simulink library "powerlib_modelsV2"  (Simulink 6.0)
settings: Solver=ode45  SolverMode=SingleTasking  StartTime=0.0  StopTime=10.0  RelTol=1e-3
values from neighbouring files (symbols this model uses):
  Ts = get(handles.edit1,'string')    [powergui.m]
undefined symbols (not defined in the file or in its folder): A, Ac, B, Bc, C, Cc, Cs, Current, damp, Dc, Dd, DiscIntNeverNeededParam, dref, dwo, exc, F, fb, gate, GH, GHd, GI, GId, GL, GLd, H, HT, hyd, ib, ib2, io, isfinite, j, K, Kd, Kg, L, Lad, Laq, lim, LIM, Ll, Llfd, Llkd, Llkq1, Llkq2, Llr, Lls, LowerFlux, N, N2, Nb, Nb2, nb_arm, p, Par_HarmoA_pu, Par_HarmoB_pu, Par_Timing_Harmo, Par_Timing_Variation, Par_Vps, Pb ... (+57)
libraries: powerlib_extras x14
(part 11 of 11)

== system powerlib_modelsV2/Discrete/asynchronous_machine/abc2qd/Rotor reference frame ==
  In1 : Inport  Port=1  LatchInput=off
  Enable : EnablePort  StatesWhenEnabling=reset
  Mux2 : Mux  Inputs=2
  Mux3 : Mux  Inputs=2
  vdr : Fcn  Expr=-sqrt3_3 * u[2]
  vds : Fcn  Expr=one_third * (2*u[5]*u[3] + (u[5]-sqrt3*u[6]) * u[4])
  vqr : Fcn  Expr=one_third * (2*u[1] + u[2])
  vqs : Fcn  Expr=one_third * (2*u[6]*u[3] + (u[6]+sqrt3*u[5]) * u[4])
  vqr,vdr : Outport  OutputWhenDisabled=reset  InitialOutput=0
  vqs,vds : Outport  Port=2  OutputWhenDisabled=reset  InitialOutput=0
  wires:
  In1/1 -> vdr/1, vds/1, vqs/1, vqr/1
  Mux3/1 -> vqr,vdr/1  "Vqr,vdr"
  vqr/1 -> Mux3/1
  vdr/1 -> Mux3/2
  Mux2/1 -> vqs,vds/1  "Vqs,vds"
  vds/1 -> Mux2/2
  vqs/1 -> Mux2/1

== system powerlib_modelsV2/Discrete/asynchronous_machine/abc2qd/Stationary reference frame ==
  In1 : Inport  Port=1  LatchInput=off
  Enable : EnablePort  StatesWhenEnabling=reset
  Mux2 : Mux  Inputs=2
  Mux3 : Mux  Inputs=2
  vdr : Fcn  Expr=one_third * (-2*u[5]*u[1] + (-u[5]-sqrt3*u[6]) * u[2])
  vds : Fcn  Expr=-sqrt3_3*u[4]
  vqr : Fcn  Expr=one_third * (2*u[6]*u[1] + (u[6]-sqrt3*u[5]) * u[2])
  vqs : Fcn  Expr=one_third * (2*u[3] + u[4])
  vqr,vdr : Outport  OutputWhenDisabled=reset  InitialOutput=0
  vqs,vds : Outport  Port=2  OutputWhenDisabled=reset  InitialOutput=0
  wires:
  Mux3/1 -> vqr,vdr/1  "Vqr,vdr"
  In1/1 -> vdr/1, vqs/1, vds/1, vqr/1
  vdr/1 -> Mux3/2
  vqr/1 -> Mux3/1
  Mux2/1 -> vqs,vds/1  "Vqs,vds"
  vqs/1 -> Mux2/1
  vds/1 -> Mux2/2

== system powerlib_modelsV2/Discrete/asynchronous_machine/abc2qd/Synchronous reference frame ==
  In1 : Inport  Port=1  LatchInput=off
  Enable : EnablePort  StatesWhenEnabling=reset
  Mux2 : Mux  Inputs=2
  Mux3 : Mux  Inputs=2
  vdr : Fcn  Expr=(2*u[5]*u[1] + (u[5]-sqrt3*u[6]) * u[2]) / 3
  vds : Fcn  Expr=(2*u[7]*u[3] + (u[7]-sqrt3*u[8]) * u[4]) / 3
  vqr : Fcn  Expr=(2*u[6]*u[1] + (u[6]+sqrt3*u[5]) * u[2]) / 3
  vqs : Fcn  Expr=(2*u[8]*u[3] + (u[8]+sqrt3*u[7]) * u[4]) / 3
  vqr,vdr : Outport  OutputWhenDisabled=reset  InitialOutput=0
  vqs,vds : Outport  Port=2  OutputWhenDisabled=reset  InitialOutput=0
  wires:
  Mux3/1 -> vqr,vdr/1  "Vqr,vdr"
  In1/1 -> vdr/1, vqs/1, vds/1, vqr/1
  vdr/1 -> Mux3/2
  vqr/1 -> Mux3/1
  Mux2/1 -> vqs,vds/1  "Vqs,vds"
  vds/1 -> Mux2/2
  vqs/1 -> Mux2/1

== system powerlib_modelsV2/Discrete/asynchronous_machine/abc2qd/transit ==
  vu : Inport  Port=1  LatchInput=off
  Constant6 : Constant  Value=[0;0]
  Mux1 : Mux  Inputs=2
  Selector : Selector  Elements=elements1  InputPortWidth=selWidth
  vr,vs : Outport
  wires:
  Selector/1 -> vr,vs/1
  vu/1 -> Mux1/2
  Mux1/1 -> Selector/1
  Constant6/1 -> Mux1/1

== system powerlib_modelsV2/Discrete/asynchronous_machine/dq2abc/Rotor reference frame ==
  In1 : Inport  Port=1  LatchInput=off
  Enable : EnablePort  StatesWhenEnabling=reset
  Mux1 : Mux  Inputs=2
  Mux2 : Mux  Inputs=2
  ira : Fcn  Expr=u[1]
  irb : Fcn  Expr=-(u[1] + sqrt3*u[2]) / 2
  isa : Fcn  Expr=u[6]*u[3]+u[5]*u[4]
  isb : Fcn  Expr=((-u[6]+sqrt3*u[5])*u[3] + (-sqrt3*u[6]-u[5])*u[4]) / 2
  ira,irb : Outport  OutputWhenDisabled=reset  InitialOutput=0
  isa,isb : Outport  Port=2  OutputWhenDisabled=reset  InitialOutput=0
  wires:
  Mux2/1 -> isa,isb/1  "isa,isb"
  Mux1/1 -> ira,irb/1  "ira,irb"
  In1/1 -> isb/1, isa/1, irb/1, ira/1
  isb/1 -> Mux2/2
  isa/1 -> Mux2/1
  irb/1 -> Mux1/2
  ira/1 -> Mux1/1

== system powerlib_modelsV2/Discrete/asynchronous_machine/dq2abc/Stationary reference frame ==
  In1 : Inport  Port=1  LatchInput=off
  Enable : EnablePort  StatesWhenEnabling=reset
  Mux1 : Mux  Inputs=2
  Mux2 : Mux  Inputs=2
  ira : Fcn  Expr=u[6]*u[1] - u[5]*u[2]
  irb : Fcn  Expr=((-u[6]-sqrt3*u[5])*u[1] + (u[5]-sqrt3*u[6])*u[2]) / 2
  isa : Fcn  Expr=u[3]
  isb : Fcn  Expr=-(u[3] + sqrt3*u[4]) / 2
  ira,irb : Outport  OutputWhenDisabled=reset  InitialOutput=0
  isa,isb : Outport  Port=2  OutputWhenDisabled=reset  InitialOutput=0
  wires:
  Mux2/1 -> isa,isb/1  "isa,isb"
  Mux1/1 -> ira,irb/1  "ira,irb"
  In1/1 -> isb/1, isa/1, irb/1, ira/1
  isb/1 -> Mux2/2
  isa/1 -> Mux2/1
  irb/1 -> Mux1/2
  ira/1 -> Mux1/1

== system powerlib_modelsV2/Discrete/asynchronous_machine/dq2abc/Synchronous reference frame ==
  In1 : Inport  Port=1  LatchInput=off
  Enable : EnablePort  StatesWhenEnabling=reset
  Mux1 : Mux  Inputs=2
  Mux2 : Mux  Inputs=2
  ira : Fcn  Expr=u[6]*u[1] + u[5]*u[2]
  irb : Fcn  Expr=((-u[6]+sqrt3*u[5])*u[1] + (-sqrt3*u[6]-u[5])*u[2]) / 2
  isa : Fcn  Expr=u[8]*u[3] + u[7]*u[4]
  isb : Fcn  Expr=((-u[8]+sqrt3*u[7])*u[3] + (-sqrt3*u[8]-u[7])*u[4]) / 2
  ira,irb : Outport  OutputWhenDisabled=reset  InitialOutput=0
  isa,isb : Outport  Port=2  OutputWhenDisabled=reset  InitialOutput=0
  wires:
  Mux2/1 -> isa,isb/1  "isa,isb"
  Mux1/1 -> ira,irb/1  "ira,irb"
  In1/1 -> isb/1, isa/1, irb/1, ira/1
  isb/1 -> Mux2/2
  isa/1 -> Mux2/1
  irb/1 -> Mux1/2
  ira/1 -> Mux1/1

== system powerlib_modelsV2/Discrete/asynchronous_machine/sin,cos/sin(beta),cos(beta),sin(th),cos(th) ==
  thr,wr : Inport  Port=1  LatchInput=off
  Enable : EnablePort  StatesWhenEnabling=reset
  Clock : Clock
      settings: Decimation=10
  Demux2 : Demux  Outputs=2
  Mux1 : Mux
  Sum : Sum  Inputs=-+|  SaturateOnIntegerOverflow=on  InputSameDT=on
  Sum1 : Sum  Inputs=|-+  SaturateOnIntegerOverflow=on  InputSameDT=on
  Trigonometric Function : Trigonometry
  Trigonometric Function1 : Trigonometry
  Trigonometric Function2 : Trigonometry  Operator=cos
  Trigonometric Function3 : Trigonometry  Operator=cos
  we : Constant
  web_psb : Gain  Gain=web_psb  SaturateOnIntegerOverflow=on
  "sin(beta),cos(beta), sin(th),cos(th)" : Outport  InitialOutput=0
  we-wr : Outport  Port=2  InitialOutput=0
  wires:
  thr,wr/1 -> Demux2/1
  Demux2/2 -> Sum/1  "wr"
  Trigonometric Function1/1 -> Mux1/1
  Trigonometric Function2/1 -> Mux1/2
  Trigonometric Function/1 -> Mux1/3
  Trigonometric Function3/1 -> Mux1/4
  Mux1/1 -> "sin(beta),cos(beta), sin(th),cos(th)"/1
  Sum1/1 -> Trigonometric Function1/1, Trigonometric Function2/1  "beta"
  Demux2/1 -> Sum1/1  "thr"
  web_psb/1 -> Sum1/2, Trigonometric Function/1, Trigonometric Function3/1  "th"
  Clock/1 -> web_psb/1
  Sum/1 -> we-wr/1  "we-wr"
  we/1 -> Sum/2

== system powerlib_modelsV2/Discrete/asynchronous_machine/sin,cos/sin(thr),cos(thr) ==
  thr : Inport  Port=1  LatchInput=off
  Enable : EnablePort  StatesWhenEnabling=reset
  Constant : Constant  Value=[0; 0]
  Mux2 : Mux  Inputs=3
  Trigonometric Function : Trigonometry
  Trigonometric Function1 : Trigonometry  Operator=cos
  sin(thr),cos(thr) : Outport  OutputWhenDisabled=reset  InitialOutput=0
  wires:
  Trigonometric Function/1 -> Mux2/1
  Trigonometric Function1/1 -> Mux2/2
  Constant/1 -> Mux2/3
  thr/1 -> Trigonometric Function/1, Trigonometric Function1/1
  Mux2/1 -> sin(thr),cos(thr)/1

== system powerlib_modelsV2/Discrete/simplified_sync_mach/Vt/LL2LN ==
  In1 : Inport  Port=1  LatchInput=off
  Enable : EnablePort
  Fcn : Fcn  Expr=(2*u(1)+u(2))/3
  Fcn1 : Fcn  Expr=(u(2)-u(1))/3
  Mux1 : Mux  Inputs=3
  Sum1 : Sum  Orientation=down  Inputs=--  SaturateOnIntegerOverflow=on  InputSameDT=on
  Out1 : Outport  OutputWhenDisabled=reset  InitialOutput=[0 0 0]
  wires:
  In1/1 -> Fcn1/1, Fcn/1
  Mux1/1 -> Out1/1
  Fcn/1 -> Mux1/1, Sum1/2
  Fcn1/1 -> Mux1/2, Sum1/1
  Sum1/1 -> Mux1/3

== system powerlib_modelsV2/Discrete/simplified_sync_mach/mechanics/Predict ==
  I : Inport  Port=1  LatchInput=off
  1\Llr4 : Gain  Gain=2  SaturateOnIntegerOverflow=on
  Sum5 : Sum  Inputs=+-  SaturateOnIntegerOverflow=on  InputSameDT=on
  Unit Delay2 : UnitDelay  X0=dwo  SampleTime=Ts
  O : Outport
  wires:
  Sum5/1 -> O/1
  I/1 -> 1\Llr4/1, Unit Delay2/1
  Unit Delay2/1 -> Sum5/2
  1\Llr4/1 -> Sum5/1

== system powerlib_modelsV2/Discrete/synchronous_machine/Delta angle/Cartesian to Polar ==
  x : Inport  Port=1  LatchInput=off
  y : Inport  Port=2  LatchInput=off
  Mux : Mux  Inputs=2
  x->r : Fcn  Expr=hypot(u[1],u[2])
  x->theta : Fcn  Expr=atan2(u[2],u[1])
  r : Outport  InitialOutput=0
  theta : Outport  Port=2  InitialOutput=0
  wires:
  Mux/1 -> x->theta/1, x->r/1
  x->r/1 -> r/1
  x/1 -> Mux/1
  y/1 -> Mux/2
  x->theta/1 -> theta/1

== system powerlib_modelsV2/Discrete/synchronous_machine/Delta angle/Radians to Degrees ==
  Radians in : Inport  Port=1  LatchInput=off
  Gain : Gain  Gain=180/pi  SaturateOnIntegerOverflow=on
  Degrees out : Outport  InitialOutput=0
  wires:
  Gain/1 -> Degrees out/1
  Radians in/1 -> Gain/1

== system powerlib_modelsV2/Discrete/synchronous_machine/currents and mutual fluxes/Saturation ==
  phimq_in : Inport  Port=1  LatchInput=off
  phimd_in : Inport  Port=2  LatchInput=off
  Data Type  Conversion{,1..4} (5 alike) : DataTypeConversion  SaturateOnIntegerOverflow=on  RndMeth=Zero
  Gain : Gain  Gain=2  SaturateOnIntegerOverflow=on
  Gain1 : Gain  Gain=3  SaturateOnIntegerOverflow=on
  Logical Operator : Logic  Operator=NOT  Inputs=1
  Logical Operator1 : Logic  Operator=NOT  Inputs=1
  Logical Operator2 : Logic
  Logical Operator3 : Logic  Orientation=down
  Multiport Switch : MultiPortSwitch  Inputs=3  InputSameDT=on
  Sum : Sum  Inputs=+++  SaturateOnIntegerOverflow=on  InputSameDT=on
  Switch : Switch  Threshold=0.5  InputSameDT=on
  Vs4 : Constant  Value=phis==1e6
  Vs5 : Constant  Value=isinf(Llkq2)
  d axis saturation : Subsystem  TreatAsAtomicUnit=on
  dq axis saturation : Subsystem  TreatAsAtomicUnit=on
  phimq_out : Outport
  phimd_out : Outport  Port=2
  wires:
  Data Type  Conversion4/1 -> Gain1/1
  Data Type  Conversion3/1 -> Logical Operator1/1, Logical Operator3/1
  Vs5/1 -> Data Type  Conversion3/1
  Data Type  Conversion2/1 -> Data Type  Conversion4/1, Logical Operator/1
  Vs4/1 -> Data Type  Conversion2/1
  Data Type  Conversion1/1 -> d axis saturation/Enable, Gain/1
  Logical Operator3/1 -> Data Type  Conversion1/1
  Data Type  Conversion/1 -> dq axis saturation/Enable, Sum/1, Switch/2
  Logical Operator2/1 -> Data Type  Conversion/1
  phimd_in/1 -> dq axis saturation/1(phimd), d axis saturation/1(phimd), Multiport Switch/4
  dq axis saturation/1(phimq sat.) -> Switch/1
  phimq_in/1 -> dq axis saturation/2(phimq), Switch/3
  Gain/1 -> Sum/2
  Sum/1 -> Multiport Switch/1
  dq axis saturation/2(phimd sat.) -> Multiport Switch/2
  d axis saturation/1(phimd sat.) -> Multiport Switch/3  "phimds"
  Gain1/1 -> Sum/3
  Logical Operator1/1 -> Logical Operator2/2
  Logical Operator/1 -> Logical Operator2/1, Logical Operator3/2
  Multiport Switch/1 -> phimd_out/1
  Switch/1 -> phimq_out/1

== system powerlib_modelsV2/Discrete/synchronous_machine/phikq2/Enabled integrator ==
  In1 : Inport  Port=1  LatchInput=off
  Enable : EnablePort
  Discrete-Time Integrator : DiscreteIntegrator  IntegratorMethod=Integration: Trapezoidal  InitialCondition=phikq2o  SampleTime=Ts  SaturateOnIntegerOverflow=on  ICPrevOutput=DiscIntNeverNeededParam  ICPrevScaledInput=DiscIntNeverNeededParam
  Out1 : Outport
  wires:
  In1/1 -> Discrete-Time Integrator/1
  Discrete-Time Integrator/1 -> Out1/1

== system powerlib_modelsV2/Phasors/Dynamic_Load/Break  Alg. Loop I1/imag ==
  In1 : Inport  Port=1  LatchInput=off
  State Space : StateSpace  A=A  B=B  C=C  D=Dd  X0=X0
  Out1 : Outport  InitialOutput=0
  wires:
  In1/1 -> State Space/1
  State Space/1 -> Out1/1

== system powerlib_modelsV2/Phasors/Dynamic_Load/Break  Alg. Loop I1/real ==
  In1 : Inport  Port=1  LatchInput=off
  State Space : StateSpace  A=A  B=B  C=C  D=Dd  X0=X0
  Out1 : Outport  InitialOutput=0
  wires:
  In1/1 -> State Space/1
  State Space/1 -> Out1/1

== system powerlib_modelsV2/Phasors/Dynamic_Load/Power/TF_P ==
  In1 : Inport  Port=1  LatchInput=off
  State-Space : StateSpace  A=Ac  B=Bc  C=Cc  D=Dc  X0=x0c
  Out1 : Outport
  wires:
  State-Space/1 -> Out1/1
  In1/1 -> State-Space/1

== system powerlib_modelsV2/Phasors/Dynamic_Load/Power/TF_Q ==
  In1 : Inport  Port=1  LatchInput=off
  State-Space : StateSpace  A=Ac  B=Bc  C=Cc  D=Dc  X0=x0c
  Out1 : Outport
  wires:
  In1/1 -> State-Space/1
  State-Space/1 -> Out1/1

== system powerlib_modelsV2/Phasors/asynchronous_machine/Negative Sequence Model/Equivalent R2 L2 ==
  s2 : Inport  Port=1  LatchInput=off
  Complex to Real-Imag : ComplexToRealImag
  Constant4 : Constant  Value=j*Lm
  Constant5 : Constant  Value=Rs+j*Lls
  Product1 : Product  Inputs=*/  SaturateOnIntegerOverflow=on  InputSameDT=on
  Product2 : Product  Inputs=**  SaturateOnIntegerOverflow=on  InputSameDT=on
  Product3 : Product  Inputs=*/  SaturateOnIntegerOverflow=on  InputSameDT=on
  Product4 : Product  Inputs=/*  SaturateOnIntegerOverflow=on  InputSameDT=on
  Sum1 : Sum  SaturateOnIntegerOverflow=on  InputSameDT=on
  Sum2 : Sum  SaturateOnIntegerOverflow=on  InputSameDT=on
  Zr : Subsystem
  L2_pu : Outport
  R2/L2_pu : Outport  Port=2
  Zm/(Zr+Zm) : Outport  Port=3
  wires:
  Product4/1 -> Zm/(Zr+Zm)/1
  Product1/1 -> R2/L2_pu/1
  Complex to Real-Imag/1 -> Product1/1
  Complex to Real-Imag/2 -> Product1/2, L2_pu/1
  Sum2/1 -> Complex to Real-Imag/1  "Z2"
  s2/1 -> Zr/1(s)
  Sum1/1 -> Product4/1, Product3/2  "Zr+Zm"
  Constant5/1 -> Sum2/2  "Zs"
  Product3/1 -> Sum2/1  "Zr//Zm"
  Constant4/1 -> Product4/2, Sum1/2, Product2/2  "Zm"
  Zr/1(Zr) -> Sum1/1, Product2/1  "Zr"
  Product2/1 -> Product3/1  "Zr*Zm"

== system powerlib_modelsV2/Phasors/asynchronous_machine/Positive Sequence Model/Mutual fluxes ==
  phiqr,phidr : Inport  Port=1  LatchInput=off
  phiqs,phids : Inport  Port=2  LatchInput=off
  1\Llr : Gain  Gain=1/Llr  SaturateOnIntegerOverflow=on
  1\Llr1 : Gain  Gain=Laq  SaturateOnIntegerOverflow=on
  1\Llr2 : Gain  Gain=Lad  SaturateOnIntegerOverflow=on
  1\Lls : Gain  Gain=1/Lls  SaturateOnIntegerOverflow=on
  Demux1 : Demux  Outputs=2
  Demux2 : Demux  Outputs=2
  Mux3 : Mux  Inputs=2
  Sum : Sum  Inputs=|++  SaturateOnIntegerOverflow=on  InputSameDT=on
  Sum1 : Sum  Inputs=++|  SaturateOnIntegerOverflow=on  InputSameDT=on
  phimq,phimd : Outport
  wires:
  Sum1/1 -> 1\Llr2/1
  phiqs,phids/1 -> 1\Lls/1
  phiqr,phidr/1 -> 1\Llr/1
  1\Llr/1 -> Demux1/1
  Demux1/1 -> Sum/1
  Sum/1 -> 1\Llr1/1
  1\Lls/1 -> Demux2/1
  Demux2/1 -> Sum/2
  Demux2/2 -> Sum1/2
  Demux1/2 -> Sum1/1
  1\Llr1/1 -> Mux3/1
  1\Llr2/1 -> Mux3/2
  Mux3/1 -> phimq,phimd/1

== system powerlib_modelsV2/Phasors/asynchronous_machine/Positive Sequence Model/Rotor ==
  vqr,vdr : Inport  Port=1  LatchInput=off
  w-wr : Inport  Port=2  LatchInput=off
  phimq,phimd : Inport  Port=3  LatchInput=off
  1\Llr : Gain  Gain=1/Llr  SaturateOnIntegerOverflow=on
  1\Llr1 : Gain  Gain=Rr  SaturateOnIntegerOverflow=on
  1\Llr2 : Gain  Gain=1/Llr  SaturateOnIntegerOverflow=on
  1\Llr3 : Gain  Gain=Rr  SaturateOnIntegerOverflow=on
  Demux : Demux  Outputs=2
  Demux1 : Demux  Outputs=2
  Mux2 : Mux  Inputs=2
  Mux3 : Mux  Inputs=2
  Product : Product  SaturateOnIntegerOverflow=on  InputSameDT=on
  Product1 : Product  Orientation=left  SaturateOnIntegerOverflow=on  InputSameDT=on
  Sum1 : Sum  Inputs=++-||  SaturateOnIntegerOverflow=on  InputSameDT=on
  Sum2 : Sum  Inputs=+--  SaturateOnIntegerOverflow=on  InputSameDT=on
  Sum3 : Sum  Inputs=+-|  SaturateOnIntegerOverflow=on  InputSameDT=on
  Sum4 : Sum  Inputs=-+|  SaturateOnIntegerOverflow=on  InputSameDT=on
  phidr : Integrator  InitialCondition=phirdo
  phiqr : Integrator  InitialCondition=phirqo
  web : Gain  Gain=web  SaturateOnIntegerOverflow=on
  web1 : Gain  Gain=web  SaturateOnIntegerOverflow=on
  iqr,idr : Outport
  phiqr,phidr : Outport  Port=2
  wires:
  phimq,phimd/1 -> Demux1/1
  Demux1/1 -> Sum3/2
  Demux/1 -> Sum2/1
  Sum3/1 -> 1\Llr/1
  1\Llr1/1 -> Sum2/3
  1\Llr/1 -> 1\Llr1/1, Mux2/1  "iqr"
  Mux2/1 -> iqr,idr/1
  Demux1/2 -> Sum4/1
  Sum4/1 -> 1\Llr2/1
  1\Llr2/1 -> Mux2/2, 1\Llr3/1  "idr"
  1\Llr3/1 -> Sum1/3
  Demux/2 -> Sum1/2
  Product1/1 -> Sum1/1
  vqr,vdr/1 -> Demux/1
  phidr/1 -> Mux3/2, Product/1, Sum4/2
  Sum2/1 -> web/1
  web/1 -> phiqr/1
  Product/1 -> Sum2/2
  w-wr/1 -> Product1/1, Product/2
  Sum1/1 -> web1/1
  web1/1 -> phidr/1
  phiqr/1 -> Sum3/1, Product1/2, Mux3/1  "phiqr"
  Mux3/1 -> phiqr,phidr/1

== system powerlib_modelsV2/Phasors/asynchronous_machine/Positive Sequence Model/Stator ==
  note: (phids - phimd)/Lls=ids
  note: Vds -Rsids +w*phiqs = web*d/dt(phids)
  note: (phiqs - phimq)/Lls=iqs
  note: Vqs -Rsiqs -w*phids = web*d/dt(phiqs)
  note: phiqs= -(Vds -Rs* ids)/w
  note: phids= (Vqs -Rs* iqs)/w
  phimq,phimd : Inport  Port=1  LatchInput=off
  vqs,vds : Inport  Port=2  LatchInput=off
  w : Inport  Port=3  LatchInput=off
  1\Llr : Gain  Gain=1/Lls  SaturateOnIntegerOverflow=on
  1\Llr1 : Gain  Gain=Rs  SaturateOnIntegerOverflow=on
  1\Llr2 : Gain  Gain=1/Lls  SaturateOnIntegerOverflow=on
  1\Llr3 : Gain  Gain=Rs  SaturateOnIntegerOverflow=on
  Demux : Demux  Outputs=2
  Demux1 : Demux  Outputs=2
  Mux2 : Mux  Inputs=2
  Mux3 : Mux  Inputs=2
  Mux4 : Mux  Inputs=2
  Product : Product  SaturateOnIntegerOverflow=on  InputSameDT=on
  Product1 : Product  SaturateOnIntegerOverflow=on  InputSameDT=on
  Sum1 : Sum  Inputs=++-||  SaturateOnIntegerOverflow=on  InputSameDT=on
  Sum2 : Sum  Inputs=--+  SaturateOnIntegerOverflow=on  InputSameDT=on
  Sum3 : Sum  Inputs=-+  SaturateOnIntegerOverflow=on  InputSameDT=on
  Sum4 : Sum  Inputs=+-|  SaturateOnIntegerOverflow=on  InputSameDT=on
  phids : Integrator  InitialCondition=phisdo
  phiqs : Integrator  InitialCondition=phisqo
  web : Gain  Gain=web  SaturateOnIntegerOverflow=on
  web1 : Gain  Gain=web  SaturateOnIntegerOverflow=on
  phiqs,phids : Outport
  iqs,ids : Outport  Port=2
  phis,is : Outport  Port=3
  wires:
  w/1 -> Product1/1, Product/1
  Demux1/1 -> Sum4/2
  phimq,phimd/1 -> Demux1/1
  Sum3/1 -> 1\Llr2/1
  Demux1/2 -> Sum3/1
  vqs,vds/1 -> Demux/1
  phiqs/1 -> Sum4/1, Product1/2, Mux3/1  "phiqs"
  web/1 -> phiqs/1
  Product/1 -> Sum2/2
  Sum2/1 -> web/1
  1\Llr1/1 -> Sum2/1
  1\Llr/1 -> 1\Llr1/1, Mux2/1  "iqs"
  Sum4/1 -> 1\Llr/1
  Mux4/1 -> phis,is/1
  Mux3/1 -> Mux4/1, phiqs,phids/1
  Product1/1 -> Sum1/1
  Demux/2 -> Sum1/2  "vds"
  phids/1 -> Mux3/2, Sum3/2, Product/2  "phids"
  Sum1/1 -> web1/1
  web1/1 -> phids/1
  1\Llr3/1 -> Sum1/3
  1\Llr2/1 -> Mux2/2, 1\Llr3/1  "ids"
  Mux2/1 -> Mux4/2, iqs,ids/1
  Demux/1 -> Sum2/3  "vqs"

== system powerlib_modelsV2/Phasors/asynchronous_machine/dq2abc/Phasors Ia Ib rotor ==
  note: Ia= I1 + I2
  note: Ib= a^2*I1 + a*I2
  note: I1
  Iqdr1 : Inport  Port=1  LatchInput=off
  I2r : Inport  Port=2  LatchInput=off
  Demux : Demux  Outputs=2
  Mux1 : Mux  Inputs=2
  Mux2 : Mux  Inputs=[2 1]
  Real-Imag to Complex : RealImagToComplex
  Sum : Sum  Orientation=down  Inputs=1  SaturateOnIntegerOverflow=on  InputSameDT=on
  Sum1 : Sum  SaturateOnIntegerOverflow=on  InputSameDT=on
  Sum3 : Sum  SaturateOnIntegerOverflow=on  InputSameDT=on
  a : Gain  Gain=exp(j*2*pi/3)  SaturateOnIntegerOverflow=on
  a^2 : Gain  Gain=exp(-j*2*pi/3)  SaturateOnIntegerOverflow=on
  inv : Gain  Gain=-1  SaturateOnIntegerOverflow=on
  Irabc cmplx : Outport
  wires:
  Real-Imag to Complex/1 -> a^2/1, Sum3/1  "I1"
  a^2/1 -> Sum1/1
  a/1 -> Sum1/2
  Sum3/1 -> Mux1/1
  Sum1/1 -> Mux1/2
  Iqdr1/1 -> Demux/1
  Mux1/1 -> Sum/1, Mux2/1  "ia ib"
  Sum/1 -> inv/1
  inv/1 -> Mux2/2  "ic"
  Mux2/1 -> Irabc cmplx/1
  Demux/1 -> Real-Imag to Complex/2
  Demux/2 -> Real-Imag to Complex/1
  I2r/1 -> Sum3/2, a/1  "I2"

== system powerlib_modelsV2/Phasors/asynchronous_machine/dq2abc/Phasors Ia Ib stator ==
  note: I1
  note: Ib= a^2*I1 + a*I2
  note: Ia= I1 + I2
  Iqds1 : Inport  Port=1  LatchInput=off
  I2s : Inport  Port=2  LatchInput=off
  Demux : Demux  Outputs=2
  Mux1 : Mux  Inputs=2
  Mux2 : Mux  Inputs=[2 1]
  Real-Imag to Complex : RealImagToComplex
  Sum : Sum  Orientation=down  Inputs=1  SaturateOnIntegerOverflow=on  InputSameDT=on
  Sum1 : Sum  SaturateOnIntegerOverflow=on  InputSameDT=on
  Sum3 : Sum  SaturateOnIntegerOverflow=on  InputSameDT=on
  a : Gain  Gain=exp(j*2*pi/3)  SaturateOnIntegerOverflow=on
  a^2 : Gain  Gain=exp(-j*2*pi/3)  SaturateOnIntegerOverflow=on
  inv : Gain  Gain=-1  SaturateOnIntegerOverflow=on
  Isabc cmplx : Outport
  wires:
  Sum3/1 -> Mux1/1
  Real-Imag to Complex/1 -> Sum3/1, a^2/1  "I1"
  I2s/1 -> a/1, Sum3/2  "I2"
  Demux/2 -> Real-Imag to Complex/1
  Demux/1 -> Real-Imag to Complex/2
  Mux2/1 -> Isabc cmplx/1
  inv/1 -> Mux2/2  "ic"
  Sum/1 -> inv/1
  Mux1/1 -> Sum/1, Mux2/1  "ia ib"
  Iqds1/1 -> Demux/1
  Sum1/1 -> Mux1/2
  a/1 -> Sum1/2
  a^2/1 -> Sum1/1

== system powerlib_modelsV2/Phasors/simplified_sync_mach/Idq1 Idq2 Pe /Vdq1->Idq1 ==
  In1 : Inport  Port=1  LatchInput=off
  Gain1 : Gain  Orientation=left  Gain=R/L  SaturateOnIntegerOverflow=on
  Gain2 : Gain  Gain=1/L  SaturateOnIntegerOverflow=on
  Gain3 : Gain  Orientation=left  Gain=[-1 1]  SaturateOnIntegerOverflow=on
  Integrator : Integrator  InitialCondition="[Id1o  Iq1o]"
  Selector1 : Selector  Orientation=left  Elements=[2 1]  InputPortWidth=2
  Sum : Sum  Inputs=+-+  SaturateOnIntegerOverflow=on  InputSameDT=on
  web : Gain  Gain=web  SaturateOnIntegerOverflow=on
  Out1 : Outport
  wires:
  Sum/1 -> web/1
  Gain2/1 -> Sum/1
  Integrator/1 -> Gain1/1, Gain3/1, Out1/1
  Gain1/1 -> Sum/2
  Gain3/1 -> Selector1/1
  Selector1/1 -> Sum/3
  In1/1 -> Gain2/1
  web/1 -> Integrator/1

== system powerlib_modelsV2/Phasors/simplified_sync_mach/Idq1 Idq2 Pe /Vdq2->Idq2 ==
  In1 : Inport  Port=1  LatchInput=off
  Gain1 : Gain  Orientation=left  Gain=R/L  SaturateOnIntegerOverflow=on
  Gain2 : Gain  Gain=1/L  SaturateOnIntegerOverflow=on
  Gain3 : Gain  Orientation=left  Gain=[-1 1]  SaturateOnIntegerOverflow=on
  Integrator : Integrator  InitialCondition=[0 0]
  Selector1 : Selector  Orientation=left  Elements=[2 1]  InputPortWidth=2
  Sum : Sum  Inputs=+-+  SaturateOnIntegerOverflow=on  InputSameDT=on
  web : Gain  Gain=web  SaturateOnIntegerOverflow=on
  Out1 : Outport
  wires:
  In1/1 -> Gain2/1
  Selector1/1 -> Sum/3
  Gain3/1 -> Selector1/1
  Gain1/1 -> Sum/2
  Integrator/1 -> Out1/1, Gain3/1, Gain1/1
  Gain2/1 -> Sum/1
  Sum/1 -> web/1
  web/1 -> Integrator/1

== system powerlib_modelsV2/Phasors/synchronous_machine/Delta angle/Cartesian to Polar ==
  x : Inport  Port=1  LatchInput=off
  y : Inport  Port=2  LatchInput=off
  Mux : Mux  Inputs=2
  x->r : Fcn  Expr=hypot(u[1],u[2])
  x->theta : Fcn  Expr=atan2(u[2],u[1])
  r : Outport  InitialOutput=0
  theta : Outport  Port=2  InitialOutput=0
  wires:
  x->theta/1 -> theta/1
  y/1 -> Mux/2
  x/1 -> Mux/1
  x->r/1 -> r/1
  Mux/1 -> x->r/1, x->theta/1

== system powerlib_modelsV2/Phasors/synchronous_machine/Delta angle/Radians to Degrees ==
  Radians in : Inport  Port=1  LatchInput=off
  Gain : Gain  Gain=180/pi  SaturateOnIntegerOverflow=on
  Degrees out : Outport  InitialOutput=0
  wires:
  Radians in/1 -> Gain/1
  Gain/1 -> Degrees out/1

== system powerlib_modelsV2/Phasors/synchronous_machine/Vd1 Vq1, I2 /Vdq2->Idq2 ==
  note: Implementation of
      | V=RI+L.dI/dt  -> dI/dt=-R/L*I  - V
      |
      | In dq components:
      | did/dt= w*(-r/l*id  +iq +vd/l)
      | diq/dt= w*(-r/l*iq -id + vq/l)
      | where r, l, i ,v are in pu
  V2_dq : Inport  Port=1  LatchInput=off
  -1/L2_pu : Gain  Gain=-1/L2_pu  SaturateOnIntegerOverflow=on
  Demux : Demux  Outputs=2
  Gain3 : Gain  Orientation=left  Gain=[-1 1]  SaturateOnIntegerOverflow=on
  Gain4 : Gain  Gain=web  SaturateOnIntegerOverflow=on
  Integrator : Integrator  InitialCondition=[0 0]
  R2_pu/L2_pu (X2/R2=30) : Gain  Orientation=left  Gain=1/30  SaturateOnIntegerOverflow=on
  Real-Imag to Complex : RealImagToComplex
  Selector1 : Selector  Orientation=left  Elements=[2 1]  InputPortWidth=2
  Sum : Sum  Inputs=+-+  SaturateOnIntegerOverflow=on  InputSameDT=on
  I2_cmplx : Outport
  wires:
  V2_dq/1 -> -1/L2_pu/1
  Selector1/1 -> Sum/3
  Gain3/1 -> Selector1/1
  R2_pu/L2_pu (X2/R2=30)/1 -> Sum/2
  Integrator/1 -> Gain3/1, R2_pu/L2_pu (X2/R2=30)/1, Demux/1  "I2_dq"
  -1/L2_pu/1 -> Sum/1
  Sum/1 -> Gain4/1
  Gain4/1 -> Integrator/1
  Demux/1 -> Real-Imag to Complex/1
  Demux/2 -> Real-Imag to Complex/2
  Real-Imag to Complex/1 -> I2_cmplx/1

== system powerlib_modelsV2/Phasors/synchronous_machine/currents and mutual fluxes/Saturation ==
  phimq_in : Inport  Port=1  LatchInput=off
  phimd_in : Inport  Port=2  LatchInput=off
  Data Type  Conversion{,1..4} (5 alike) : DataTypeConversion  SaturateOnIntegerOverflow=on  RndMeth=Zero
  Gain : Gain  Gain=2  SaturateOnIntegerOverflow=on
  Gain1 : Gain  Gain=3  SaturateOnIntegerOverflow=on
  Logical Operator : Logic  Operator=NOT  Inputs=1
  Logical Operator1 : Logic  Operator=NOT  Inputs=1
  Logical Operator2 : Logic
  Logical Operator3 : Logic  Orientation=down
  Multiport Switch : MultiPortSwitch  Inputs=3  InputSameDT=on
  Sum : Sum  Inputs=+++  SaturateOnIntegerOverflow=on  InputSameDT=on
  Switch : Switch  Threshold=0.5  InputSameDT=on
  Vs4 : Constant  Value=phis==1e6
  Vs5 : Constant  Value=isinf(Llkq2)
  d axis saturation : Subsystem  TreatAsAtomicUnit=on
  dq axis saturation : Subsystem  TreatAsAtomicUnit=on
  phimq_out : Outport
  phimd_out : Outport  Port=2
  wires:
  Data Type  Conversion4/1 -> Gain1/1
  Data Type  Conversion3/1 -> Logical Operator3/1, Logical Operator1/1
  Vs5/1 -> Data Type  Conversion3/1
  Data Type  Conversion1/1 -> Gain/1, d axis saturation/Enable
  Logical Operator3/1 -> Data Type  Conversion1/1
  Data Type  Conversion/1 -> Switch/2, Sum/1, dq axis saturation/Enable
  Logical Operator2/1 -> Data Type  Conversion/1
  Switch/1 -> phimq_out/1
  Multiport Switch/1 -> phimd_out/1
  Logical Operator/1 -> Logical Operator3/2, Logical Operator2/1
  Logical Operator1/1 -> Logical Operator2/2
  Gain1/1 -> Sum/3
  d axis saturation/1(phimd sat.) -> Multiport Switch/3  "phimds"
  dq axis saturation/2(phimd sat.) -> Multiport Switch/2
  Sum/1 -> Multiport Switch/1
  Gain/1 -> Sum/2
  phimq_in/1 -> Switch/3, dq axis saturation/2(phimq)
  dq axis saturation/1(phimq sat.) -> Switch/1
  phimd_in/1 -> Multiport Switch/4, d axis saturation/1(phimd), dq axis saturation/1(phimd)
  Data Type  Conversion2/1 -> Logical Operator/1
  Vs4/1 -> Data Type  Conversion2/1, Data Type  Conversion4/1

== system powerlib_modelsV2/Phasors/synchronous_machine/phikq2/Enabled integrator ==
  In1 : Inport  Port=1  LatchInput=off
  Enable : EnablePort
  int : Integrator  InitialCondition=phikq2o
  Out1 : Outport  InitialOutput=phikq2o
  wires:
  int/1 -> Out1/1
  In1/1 -> int/1

== system powerlib_modelsV2/Switch Current Source/IGBT/Conduction Logic/Break Alg. Loop ==
  In1 : Inport  Port=1  LatchInput=off
  0 2 : Constant  Value=0.001
  Data Type  Conversion : DataTypeConversion  SaturateOnIntegerOverflow=on  RndMeth=Zero
  Data Type  Conversion1 : DataTypeConversion  SaturateOnIntegerOverflow=on  RndMeth=Zero
  Integrator : Integrator  LimitOutput=on  UpperSaturationLimit=0.00101
  R_device : Gain  Gain=1e7  SaturateOnIntegerOverflow=on
  Relational Operator1 : RelationalOperator  Operator=>  InputSameDT=on
  Vak-Vf-Ron*Iak : Sum  Inputs=+-  SaturateOnIntegerOverflow=on  InputSameDT=on
  Out1 : Outport
  wires:
  Relational Operator1/1 -> Data Type  Conversion/1
  0 2/1 -> Relational Operator1/2
  Integrator/1 -> Relational Operator1/1, Vak-Vf-Ron*Iak/2
  Vak-Vf-Ron*Iak/1 -> R_device/1
  R_device/1 -> Integrator/1
  Data Type  Conversion1/1 -> Vak-Vf-Ron*Iak/1
  In1/1 -> Data Type  Conversion1/1
  Data Type  Conversion/1 -> Out1/1

== system powerlib_modelsV2/Switch Current Source/detailed_thyristor/Conduction logic/Break Alg. Loop ==
  In1 : Inport  Port=1  LatchInput=off
  0 2 : Constant  Value=0.001
  Data Type  Conversion1 : DataTypeConversion  SaturateOnIntegerOverflow=on  RndMeth=Zero
  Data Type  Conversion2 : DataTypeConversion  SaturateOnIntegerOverflow=on  RndMeth=Zero
  Integrator : Integrator  InitialCondition=0.00101*(IC&1)  LimitOutput=on  UpperSaturationLimit=0.00101
  R_device : Gain  Gain=1e7  SaturateOnIntegerOverflow=on
  Relational Operator1 : RelationalOperator  Operator=>  InputSameDT=on
  Vak-Vf-Ron*Iak : Sum  Inputs=+-  SaturateOnIntegerOverflow=on  InputSameDT=on
  Out1 : Outport
  wires:
  Data Type  Conversion2/1 -> Out1/1
  Relational Operator1/1 -> Data Type  Conversion2/1
  0 2/1 -> Relational Operator1/2
  Integrator/1 -> Relational Operator1/1, Vak-Vf-Ron*Iak/2
  Vak-Vf-Ron*Iak/1 -> R_device/1
  R_device/1 -> Integrator/1
  Data Type  Conversion1/1 -> Vak-Vf-Ron*Iak/1
  In1/1 -> Data Type  Conversion1/1

== system powerlib_modelsV2/Switch Current Source/detailed_thyristor/Conduction logic/Time recovery ==
  Iak>0 : Inport  Port=1  LatchInput=off
  "Vak>Vf " : Inport  Port=2  LatchInput=off
  Iak>il : Inport  Port=3  LatchInput=off
  Data Type  Conversion : DataTypeConversion  SaturateOnIntegerOverflow=on  RndMeth=Zero
  Data Type  Conversion1 : DataTypeConversion  SaturateOnIntegerOverflow=on  RndMeth=Zero
  Product : Product  SaturateOnIntegerOverflow=on  InputSameDT=on
  Sum : Sum  SaturateOnIntegerOverflow=on  InputSameDT=on
  Sum1 : Sum  SaturateOnIntegerOverflow=on  InputSameDT=on
  Tq : Subsystem
  "confirmation de i>i_latching apres reamorcage, car vak peut devenir negatif  , ig etant nul, on retourne en pilotage par iak" : Relay  OnSwitchValue=1.5  OffSwitchValue=0
  "TQ " : Outport  InitialOutput=0
  wires:
  Iak>il/1 -> Sum/1
  Product/1 -> Sum1/2, Sum/2
  Iak>0/1 -> Tq/1("Iak>0 ")
  Sum/1 -> "confirmation de i>i_latching apres reamorcage, car vak peut devenir negatif  , ig etant nul, on retourne en pilotage par iak"/1
  "confirmation de i>i_latching apres reamorcage, car vak peut devenir negatif  , ig etant nul, on retourne en pilotage par iak"/1 -> Sum1/1
  Sum1/1 -> "TQ "/1
  Tq/1(out) -> Data Type  Conversion/1
  Data Type  Conversion/1 -> Product/1
  "Vak>Vf "/1 -> Data Type  Conversion1/1
  Data Type  Conversion1/1 -> Product/2

== system powerlib_modelsV2/Switch Current Source/detailed_thyristor/Conduction logic/Vak>Vf ==
  Vak : Inport  Port=1  LatchInput=off
  "  " : RelationalOperator  Operator=>  InputSameDT=on
  "Vf " : Constant  Value=Vf
  Vak>Vf : Outport  InitialOutput=0
  wires:
  "  "/1 -> Vak>Vf/1
  "Vf "/1 -> "  "/2
  Vak/1 -> "  "/1

== system powerlib_modelsV2/Switch Current Source/diode/Conduction logic/Break Alg. Loop ==
  In1 : Inport  Port=1  LatchInput=off
  0 2 : Constant  Value=0.001
  Data Type  Conversion1 : DataTypeConversion  SaturateOnIntegerOverflow=on  RndMeth=Zero
  Integrator : Integrator  InitialCondition=0.00101*(IC&1)  LimitOutput=on  UpperSaturationLimit=0.00101
  R_device : Gain  Gain=1e7  SaturateOnIntegerOverflow=on
  Relational Operator1 : RelationalOperator  Operator=>  InputSameDT=on
  Vak-Vf-Ron*Iak : Sum  Inputs=+-  SaturateOnIntegerOverflow=on  InputSameDT=on
  Out1 : Outport
  wires:
  In1/1 -> Data Type  Conversion1/1
  Data Type  Conversion1/1 -> Vak-Vf-Ron*Iak/1
  R_device/1 -> Integrator/1
  Vak-Vf-Ron*Iak/1 -> R_device/1
  Integrator/1 -> Vak-Vf-Ron*Iak/2, Relational Operator1/1
  0 2/1 -> Relational Operator1/2
  Relational Operator1/1 -> Out1/1

== system powerlib_modelsV2/Switch Current Source/gto/Conduction Logic/Break Alg. Loop ==
  In1 : Inport  Port=1  LatchInput=off
  0 2 : Constant  Value=0.001
  Data Type  Conversion : DataTypeConversion  SaturateOnIntegerOverflow=on  RndMeth=Zero
  Data Type  Conversion1 : DataTypeConversion  SaturateOnIntegerOverflow=on  RndMeth=Zero
  Integrator : Integrator  LimitOutput=on  UpperSaturationLimit=0.002  LowerSaturationLimit=0
  R_device : Gain  Gain=1e7  SaturateOnIntegerOverflow=on
  Relational Operator1 : RelationalOperator  Operator=>  InputSameDT=on
  Vak-Vf-Ron*Iak : Sum  Inputs=+-  SaturateOnIntegerOverflow=on  InputSameDT=on
  Out1 : Outport
  wires:
  Relational Operator1/1 -> Data Type  Conversion/1
  0 2/1 -> Relational Operator1/2
  Integrator/1 -> Relational Operator1/1, Vak-Vf-Ron*Iak/2
  Vak-Vf-Ron*Iak/1 -> R_device/1
  R_device/1 -> Integrator/1
  Data Type  Conversion1/1 -> Vak-Vf-Ron*Iak/1
  In1/1 -> Data Type  Conversion1/1
  Data Type  Conversion/1 -> Out1/1

== system powerlib_modelsV2/Switch Current Source/mosfet/Conduction Logic/Break Alg. Loop ==
  In1 : Inport  Port=1  LatchInput=off
  0 2 : Constant  Value=0.001
  Data Type  Conversion : DataTypeConversion  SaturateOnIntegerOverflow=on  RndMeth=Zero
  Data Type  Conversion1 : DataTypeConversion  SaturateOnIntegerOverflow=on  RndMeth=Zero
  Integrator : Integrator  LimitOutput=on  UpperSaturationLimit=0.00101
  R_device : Gain  Gain=1e7  SaturateOnIntegerOverflow=on
  Relational Operator1 : RelationalOperator  Operator=>  InputSameDT=on
  Vak-Vf-Ron*Iak : Sum  Inputs=+-  SaturateOnIntegerOverflow=on  InputSameDT=on
  Out1 : Outport
  wires:
  Relational Operator1/1 -> Data Type  Conversion/1
  0 2/1 -> Relational Operator1/2
  Integrator/1 -> Relational Operator1/1, Vak-Vf-Ron*Iak/2
  Vak-Vf-Ron*Iak/1 -> R_device/1
  R_device/1 -> Integrator/1
  Data Type  Conversion1/1 -> Vak-Vf-Ron*Iak/1
  In1/1 -> Data Type  Conversion1/1
  Data Type  Conversion/1 -> Out1/1

== system powerlib_modelsV2/Switch Current Source/thyristor/Conduction Logic/Break Alg. Loop ==
  In1 : Inport  Port=1  LatchInput=off
  0 2 : Constant  Value=0.001
  Data Type  Conversion1 : DataTypeConversion  SaturateOnIntegerOverflow=on  RndMeth=Zero
  Data Type  Conversion2 : DataTypeConversion  SaturateOnIntegerOverflow=on  RndMeth=Zero
  Integrator : Integrator  InitialCondition=0.00101*(IC&1)  LimitOutput=on  UpperSaturationLimit=0.00101
  R_device : Gain  Gain=1e7  SaturateOnIntegerOverflow=on
  Relational Operator1 : RelationalOperator  Operator=>  InputSameDT=on
  Vak-Vf-Ron*Iak : Sum  Inputs=+-  SaturateOnIntegerOverflow=on  InputSameDT=on
  Out1 : Outport
  wires:
  In1/1 -> Data Type  Conversion1/1
  Data Type  Conversion1/1 -> Vak-Vf-Ron*Iak/1
  R_device/1 -> Integrator/1
  Vak-Vf-Ron*Iak/1 -> R_device/1
  Integrator/1 -> Vak-Vf-Ron*Iak/2, Relational Operator1/1
  0 2/1 -> Relational Operator1/2
  Relational Operator1/1 -> Data Type  Conversion2/1
  Data Type  Conversion2/1 -> Out1/1

== system powerlib_modelsV2/Continuous/Three-Level Bridge/2-level GTO-IGBT Bridge  Logic (modified)/Diode Logic/Blocking Diodes ==
  G : Inport  Port=1  LatchInput=off
  Bloque D214365 : Selector  Elements=Selec_Diode  InputPortWidth=nb_switch
  Logical Operator : Logic  Operator=NOT
  Memory : Memory
  Pulse 1 step : Logic
  Block.D : Outport
  wires:
  G/1 -> Memory/1, Pulse 1 step/2
  Logical Operator/1 -> Pulse 1 step/1
  Memory/1 -> Logical Operator/1
  Pulse 1 step/1 -> Bloque D214365/1  "Blockinkg"
  Bloque D214365/1 -> Block.D/1

== system powerlib_modelsV2/Continuous/synchronous_machine/currents and mutual fluxes/Saturation/d axis saturation ==
  phimd : Inport  Port=1  LatchInput=off
  Enable : EnablePort
  Lad\Lmd : Gain  Gain=Lad/Lmd  SaturateOnIntegerOverflow=on
  Relational Operator : RelationalOperator  Operator=>  InputSameDT=on
  Sum21 : Sum  Inputs=|-+  SaturateOnIntegerOverflow=on  InputSameDT=on
  Switch : Switch  Threshold=0.5  InputSameDT=on
  Vs : Constant  Value=phis
  polynomial approximation of exp : Fcn  Expr=((((a5*u+a4)*u+a3)*u+a2)*u+a1)*u+a0
  phimd sat. : Outport  InitialOutput=0
  wires:
  Vs/1 -> Relational Operator/2
  Relational Operator/1 -> Switch/2
  Sum21/1 -> Switch/1
  polynomial approximation of exp/1 -> Lad\Lmd/1  "f(phimd)"
  Lad\Lmd/1 -> Sum21/1
  Switch/1 -> phimd sat./1
  phimd/1 -> Switch/3, polynomial approximation of exp/1, Sum21/2, Relational Operator/1

== system powerlib_modelsV2/Continuous/synchronous_machine/currents and mutual fluxes/Saturation/dq axis saturation ==
  phimd : Inport  Port=1  LatchInput=off
  phimq : Inport  Port=2  LatchInput=off
  Enable : EnablePort
  Lad\Lmd : Gain  Gain=Lad/Lmd  SaturateOnIntegerOverflow=on
  Laq\Lmq : Gain  Gain=Laq/Lmq  SaturateOnIntegerOverflow=on
  Product{,1..3} (4 alike) : Product  SaturateOnIntegerOverflow=on  InputSameDT=on
  Relational Operator : RelationalOperator  Operator=>  InputSameDT=on
  Sum : Sum  SaturateOnIntegerOverflow=on  InputSameDT=on
  Sum1 : Sum  Inputs=+-  SaturateOnIntegerOverflow=on  InputSameDT=on
  Sum2 : Sum  Inputs=-+  SaturateOnIntegerOverflow=on  InputSameDT=on
  Switch : Switch  Threshold=0.5  InputSameDT=on
  Switch1 : Switch  Threshold=0.5  InputSameDT=on
  Vs : Constant  Value=phis^2
  polynomial approximation of exp : Fcn  Expr=((((a5*u+a4)*u+a3)*u+a2)*u+a1)*u+a0
  phimq sat. : Outport  OutputWhenDisabled=reset  InitialOutput=0
  phimd sat. : Outport  Port=2  OutputWhenDisabled=reset  InitialOutput=0
  wires:
  Switch/1 -> phimd sat./1
  Switch1/1 -> phimq sat./1
  Vs/1 -> Relational Operator/2
  Relational Operator/1 -> Switch1/2, Switch/2
  Sum2/1 -> Switch1/1
  Sum1/1 -> Switch/1
  Sum/1 -> Relational Operator/1, polynomial approximation of exp/1
  Laq\Lmq/1 -> Sum2/1
  Lad\Lmd/1 -> Sum1/2
  Product3/1 -> Laq\Lmq/1  "f(phimq)"
  Product2/1 -> Lad\Lmd/1  "f(phimd)"
  polynomial approximation of exp/1 -> Product3/1, Product2/2
  Product1/1 -> Sum/2
  phimq/1 -> Switch1/3, Sum2/2, Product3/2, Product1/2, Product1/1
  Product/1 -> Sum/1
  phimd/1 -> Switch/3, Sum1/1, Product2/1, Product/2, Product/1

== system powerlib_modelsV2/Discrete/HTG/servo-motor/servo-motor/1st order Lowpass ==
  In : Inport  Port=1  LatchInput=off
  Discrete State-Space : DiscreteStateSpace  A=Ad  B=Bd  C=Cd  D=Dd  X0=x0d  SampleTime=Ts
  Out : Outport  InitialOutput=0
  wires:
  Discrete State-Space/1 -> Out/1
  In/1 -> Discrete State-Space/1

== system powerlib_modelsV2/Discrete/MBPSS/Transfer function for detailed model (HF)/Transfer functions for detailed stabilizer/Discrete Lead-Lag1 ==
  In1 : Inport  Port=1  LatchInput=off
  Discrete State-Space : DiscreteStateSpace  A=Ad  B=Bd  C=Cd  D=Dd  SampleTime=Ts
  Out1 : Outport
  wires:
  In1/1 -> Discrete State-Space/1
  Discrete State-Space/1 -> Out1/1

== system powerlib_modelsV2/Discrete/MBPSS/Transfer function for detailed model (HF)/Transfer functions for detailed stabilizer/Discrete Lead-Lag2 ==
  In1 : Inport  Port=1  LatchInput=off
  Discrete State-Space : DiscreteStateSpace  A=Ad  B=Bd  C=Cd  D=Dd  SampleTime=Ts
  Out1 : Outport
  wires:
  Discrete State-Space/1 -> Out1/1
  In1/1 -> Discrete State-Space/1

== system powerlib_modelsV2/Discrete/MBPSS/Transfer function for detailed model (HF)/Transfer functions for detailed stabilizer1/Discrete Lead-Lag1 ==
  In1 : Inport  Port=1  LatchInput=off
  Discrete State-Space : DiscreteStateSpace  A=Ad  B=Bd  C=Cd  D=Dd  SampleTime=Ts
  Out1 : Outport
  wires:
  Discrete State-Space/1 -> Out1/1
  In1/1 -> Discrete State-Space/1

== system powerlib_modelsV2/Discrete/MBPSS/Transfer function for detailed model (HF)/Transfer functions for detailed stabilizer1/Discrete Lead-Lag2 ==
  In1 : Inport  Port=1  LatchInput=off
  Discrete State-Space : DiscreteStateSpace  A=Ad  B=Bd  C=Cd  D=Dd  SampleTime=Ts
  Out1 : Outport
  wires:
  In1/1 -> Discrete State-Space/1
  Discrete State-Space/1 -> Out1/1

== system powerlib_modelsV2/Discrete/MBPSS/Transfer function for detailed model (IF)/Transfer functions for detailed stabilizer/Discrete Lead-Lag1 ==
  In1 : Inport  Port=1  LatchInput=off
  Discrete State-Space : DiscreteStateSpace  A=Ad  B=Bd  C=Cd  D=Dd  SampleTime=Ts
  Out1 : Outport
  wires:
  Discrete State-Space/1 -> Out1/1
  In1/1 -> Discrete State-Space/1

== system powerlib_modelsV2/Discrete/MBPSS/Transfer function for detailed model (IF)/Transfer functions for detailed stabilizer/Discrete Lead-Lag2 ==
  In1 : Inport  Port=1  LatchInput=off
  Discrete State-Space : DiscreteStateSpace  A=Ad  B=Bd  C=Cd  D=Dd  SampleTime=Ts
  Out1 : Outport
  wires:
  In1/1 -> Discrete State-Space/1
  Discrete State-Space/1 -> Out1/1

== system powerlib_modelsV2/Discrete/MBPSS/Transfer function for detailed model (IF)/Transfer functions for detailed stabilizer1/Discrete Lead-Lag1 ==
  In1 : Inport  Port=1  LatchInput=off
  Discrete State-Space : DiscreteStateSpace  A=Ad  B=Bd  C=Cd  D=Dd  SampleTime=Ts
  Out1 : Outport
  wires:
  In1/1 -> Discrete State-Space/1
  Discrete State-Space/1 -> Out1/1

== system powerlib_modelsV2/Discrete/MBPSS/Transfer function for detailed model (IF)/Transfer functions for detailed stabilizer1/Discrete Lead-Lag2 ==
  In1 : Inport  Port=1  LatchInput=off
  Discrete State-Space : DiscreteStateSpace  A=Ad  B=Bd  C=Cd  D=Dd  SampleTime=Ts
  Out1 : Outport
  wires:
  Discrete State-Space/1 -> Out1/1
  In1/1 -> Discrete State-Space/1

== system powerlib_modelsV2/Discrete/MBPSS/Transfer function for detailed model (LF)/Transfer functions for detailed stabilizer/Discrete Lead-Lag1 ==
  In1 : Inport  Port=1  LatchInput=off
  Discrete State-Space : DiscreteStateSpace  A=Ad  B=Bd  C=Cd  D=Dd  SampleTime=Ts
  Out1 : Outport
  wires:
  In1/1 -> Discrete State-Space/1
  Discrete State-Space/1 -> Out1/1

== system powerlib_modelsV2/Discrete/MBPSS/Transfer function for detailed model (LF)/Transfer functions for detailed stabilizer/Discrete Lead-Lag2 ==
  In1 : Inport  Port=1  LatchInput=off
  Discrete State-Space : DiscreteStateSpace  A=Ad  B=Bd  C=Cd  D=Dd  SampleTime=Ts
  Out1 : Outport
  wires:
  Discrete State-Space/1 -> Out1/1
  In1/1 -> Discrete State-Space/1

== system powerlib_modelsV2/Discrete/MBPSS/Transfer function for detailed model (LF)/Transfer functions for detailed stabilizer1/Discrete Lead-Lag1 ==
  In1 : Inport  Port=1  LatchInput=off
  Discrete State-Space : DiscreteStateSpace  A=Ad  B=Bd  C=Cd  D=Dd  SampleTime=Ts
  Out1 : Outport
  wires:
  Discrete State-Space/1 -> Out1/1
  In1/1 -> Discrete State-Space/1

== system powerlib_modelsV2/Discrete/MBPSS/Transfer function for detailed model (LF)/Transfer functions for detailed stabilizer1/Discrete Lead-Lag2 ==
  In1 : Inport  Port=1  LatchInput=off
  Discrete State-Space : DiscreteStateSpace  A=Ad  B=Bd  C=Cd  D=Dd  SampleTime=Ts
  Out1 : Outport
  wires:
  In1/1 -> Discrete State-Space/1
  Discrete State-Space/1 -> Out1/1

== system powerlib_modelsV2/Discrete/Three-Level Bridge/2-level GTO-IGBT Bridge  Logic (modified)/Diode Logic/Blocking Diodes ==
  G : Inport  Port=1  LatchInput=off
  Bloque D214365 : Selector  Elements=Selec_Diode  InputPortWidth=nb_switch
  Logical Operator : Logic  Operator=NOT
  Pulse 1 step : Logic
  Unit Delay : UnitDelay  SampleTime=Ts
  Block.D : Outport
  wires:
  Bloque D214365/1 -> Block.D/1
  Pulse 1 step/1 -> Bloque D214365/1  "Blockinkg"
  Unit Delay/1 -> Logical Operator/1
  Logical Operator/1 -> Pulse 1 step/1
  G/1 -> Unit Delay/1, Pulse 1 step/2

== system powerlib_modelsV2/Discrete/synchronous_machine/currents and mutual fluxes/Saturation/d axis saturation ==
  phimd : Inport  Port=1  LatchInput=off
  Enable : EnablePort
  Lad\Lmd : Gain  Gain=Lad/Lmd  SaturateOnIntegerOverflow=on
  Relational Operator : RelationalOperator  Operator=>  InputSameDT=on
  Sum21 : Sum  Inputs=|-+  SaturateOnIntegerOverflow=on  InputSameDT=on
  Switch : Switch  Threshold=0.5  InputSameDT=on
  Vs : Constant  Value=phis
  polynomial approximation of exp : Fcn  Expr=((((a5*u+a4)*u+a3)*u+a2)*u+a1)*u+a0
  phimd sat. : Outport  InitialOutput=0
  wires:
  phimd/1 -> Relational Operator/1, Sum21/2, polynomial approximation of exp/1, Switch/3
  Switch/1 -> phimd sat./1
  Lad\Lmd/1 -> Sum21/1
  polynomial approximation of exp/1 -> Lad\Lmd/1  "f(phimd)"
  Sum21/1 -> Switch/1
  Relational Operator/1 -> Switch/2
  Vs/1 -> Relational Operator/2

== system powerlib_modelsV2/Discrete/synchronous_machine/currents and mutual fluxes/Saturation/dq axis saturation ==
  phimd : Inport  Port=1  LatchInput=off
  phimq : Inport  Port=2  LatchInput=off
  Enable : EnablePort
  Lad\Lmd : Gain  Gain=Lad/Lmd  SaturateOnIntegerOverflow=on
  Laq\Lmq : Gain  Gain=Laq/Lmq  SaturateOnIntegerOverflow=on
  Product{,1..3} (4 alike) : Product  SaturateOnIntegerOverflow=on  InputSameDT=on
  Relational Operator : RelationalOperator  Operator=>  InputSameDT=on
  Sum : Sum  SaturateOnIntegerOverflow=on  InputSameDT=on
  Sum1 : Sum  Inputs=+-  SaturateOnIntegerOverflow=on  InputSameDT=on
  Sum2 : Sum  Inputs=-+  SaturateOnIntegerOverflow=on  InputSameDT=on
  Switch : Switch  Threshold=0.5  InputSameDT=on
  Switch1 : Switch  Threshold=0.5  InputSameDT=on
  Vs : Constant  Value=phis^2
  polynomial approximation of exp : Fcn  Expr=((((a5*u+a4)*u+a3)*u+a2)*u+a1)*u+a0
  phimq sat. : Outport  OutputWhenDisabled=reset  InitialOutput=0
  phimd sat. : Outport  Port=2  OutputWhenDisabled=reset  InitialOutput=0
  wires:
  phimd/1 -> Product/1, Product/2, Product2/1, Sum1/1, Switch/3
  Product/1 -> Sum/1
  phimq/1 -> Product1/1, Product1/2, Product3/2, Sum2/2, Switch1/3
  Product1/1 -> Sum/2
  polynomial approximation of exp/1 -> Product2/2, Product3/1
  Product2/1 -> Lad\Lmd/1  "f(phimd)"
  Product3/1 -> Laq\Lmq/1  "f(phimq)"
  Lad\Lmd/1 -> Sum1/2
  Laq\Lmq/1 -> Sum2/1
  Sum/1 -> polynomial approximation of exp/1, Relational Operator/1
  Sum1/1 -> Switch/1
  Sum2/1 -> Switch1/1
  Relational Operator/1 -> Switch/2, Switch1/2
  Vs/1 -> Relational Operator/2
  Switch1/1 -> phimq sat./1
  Switch/1 -> phimd sat./1

== system powerlib_modelsV2/Phasors/asynchronous_machine/Negative Sequence Model/Equivalent R2 L2/Zr ==
  s : Inport  Port=1  LatchInput=off
  Constant2 : Constant  Value=Rr
  Constant4 : Constant  Value=j*Llr
  Product2 : Product  Inputs=*/  SaturateOnIntegerOverflow=on  InputSameDT=on
  Sum2 : Sum  SaturateOnIntegerOverflow=on  InputSameDT=on
  Zr : Outport
  wires:
  Constant2/1 -> Product2/1
  Product2/1 -> Sum2/1
  Constant4/1 -> Sum2/2
  s/1 -> Product2/2
  Sum2/1 -> Zr/1

== system powerlib_modelsV2/Phasors/synchronous_machine/currents and mutual fluxes/Saturation/d axis saturation ==
  phimd : Inport  Port=1  LatchInput=off
  Enable : EnablePort
  Lad\Lmd : Gain  Gain=Lad/Lmd  SaturateOnIntegerOverflow=on
  Relational Operator : RelationalOperator  Operator=>  InputSameDT=on
  Sum21 : Sum  Inputs=|-+  SaturateOnIntegerOverflow=on  InputSameDT=on
  Switch : Switch  Threshold=0.5  InputSameDT=on
  Vs : Constant  Value=phis
  polynomial approximation of exp : Fcn  Expr=((((a5*u+a4)*u+a3)*u+a2)*u+a1)*u+a0
  phimd sat. : Outport  InitialOutput=0
  wires:
  Vs/1 -> Relational Operator/2
  Relational Operator/1 -> Switch/2
  Sum21/1 -> Switch/1
  polynomial approximation of exp/1 -> Lad\Lmd/1  "f(phimd)"
  Lad\Lmd/1 -> Sum21/1
  Switch/1 -> phimd sat./1
  phimd/1 -> Switch/3, polynomial approximation of exp/1, Sum21/2, Relational Operator/1

== system powerlib_modelsV2/Phasors/synchronous_machine/currents and mutual fluxes/Saturation/dq axis saturation ==
  phimd : Inport  Port=1  LatchInput=off
  phimq : Inport  Port=2  LatchInput=off
  Enable : EnablePort
  Lad\Lmd : Gain  Gain=Lad/Lmd  SaturateOnIntegerOverflow=on
  Laq\Lmq : Gain  Gain=Laq/Lmq  SaturateOnIntegerOverflow=on
  Product{,1..3} (4 alike) : Product  SaturateOnIntegerOverflow=on  InputSameDT=on
  Relational Operator : RelationalOperator  Operator=>  InputSameDT=on
  Sum : Sum  SaturateOnIntegerOverflow=on  InputSameDT=on
  Sum1 : Sum  Inputs=+-  SaturateOnIntegerOverflow=on  InputSameDT=on
  Sum2 : Sum  Inputs=-+  SaturateOnIntegerOverflow=on  InputSameDT=on
  Switch : Switch  Threshold=0.5  InputSameDT=on
  Switch1 : Switch  Threshold=0.5  InputSameDT=on
  Vs : Constant  Value=phis^2
  polynomial approximation of exp : Fcn  Expr=((((a5*u+a4)*u+a3)*u+a2)*u+a1)*u+a0
  phimq sat. : Outport  OutputWhenDisabled=reset  InitialOutput=0
  phimd sat. : Outport  Port=2  OutputWhenDisabled=reset  InitialOutput=0
  wires:
  Switch/1 -> phimd sat./1
  Switch1/1 -> phimq sat./1
  Vs/1 -> Relational Operator/2
  Relational Operator/1 -> Switch1/2, Switch/2
  Sum2/1 -> Switch1/1
  Sum1/1 -> Switch/1
  Sum/1 -> Relational Operator/1, polynomial approximation of exp/1
  Laq\Lmq/1 -> Sum2/1
  Lad\Lmd/1 -> Sum1/2
  Product3/1 -> Laq\Lmq/1  "f(phimq)"
  Product2/1 -> Lad\Lmd/1  "f(phimd)"
  polynomial approximation of exp/1 -> Product3/1, Product2/2
  Product1/1 -> Sum/2
  phimq/1 -> Switch1/3, Sum2/2, Product3/2, Product1/2, Product1/1
  Product/1 -> Sum/1
  phimd/1 -> Switch/3, Sum1/1, Product2/1, Product/2, Product/1

== system powerlib_modelsV2/Switch Current Source/detailed_thyristor/Conduction logic/Time recovery/Tq ==
  "Iak>0 " : Inport  Port=1  LatchInput=off
  . : Logic  Operator=NOT  Inputs=1
  ". " : Logic  Inputs=3
  0 : Constant  Value=0
  Data Type  Conversion{1..4} (4 alike) : DataTypeConversion  SaturateOnIntegerOverflow=on  RndMeth=Zero
  Relational Operator : RelationalOperator  Operator=<=  InputSameDT=on
  Step : Step  Time=1.1*Tq  SampleTime=0
  Transport Delay=Tq : TransportDelay  DelayTime=Tq+eps  BufferSize=2048
  out : Outport  InitialOutput=0
  wires:
  "Iak>0 "/1 -> Relational Operator/1
  0/1 -> Relational Operator/2
  ./1 -> ". "/1
  ". "/1 -> out/1
  Step/1 -> Data Type  Conversion1/1
  Data Type  Conversion1/1 -> ". "/3
  Transport Delay=Tq/1 -> Data Type  Conversion2/1
  Data Type  Conversion2/1 -> ./1
  Data Type  Conversion3/1 -> ". "/2
  Relational Operator/1 -> Data Type  Conversion4/1
  Data Type  Conversion4/1 -> Transport Delay=Tq/1, Data Type  Conversion3/1
